simulink model "fadec_limit_logic"  (R2025b)
settings: Solver=FixedStepDiscrete  StartTime=0.0  StopTime=10.0  FixedStep=0.02  RelTol=1e-3

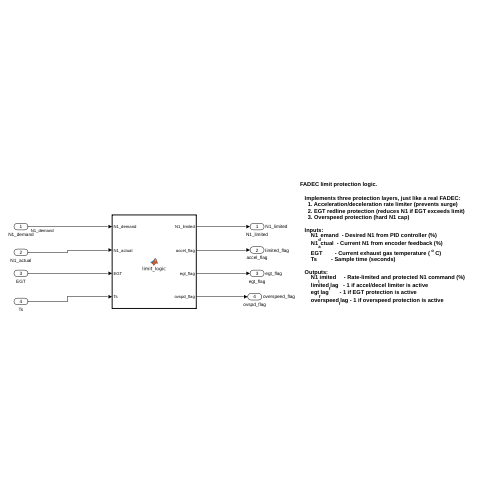
[thumbnail: Simulink's stored preview of the top-level diagram]
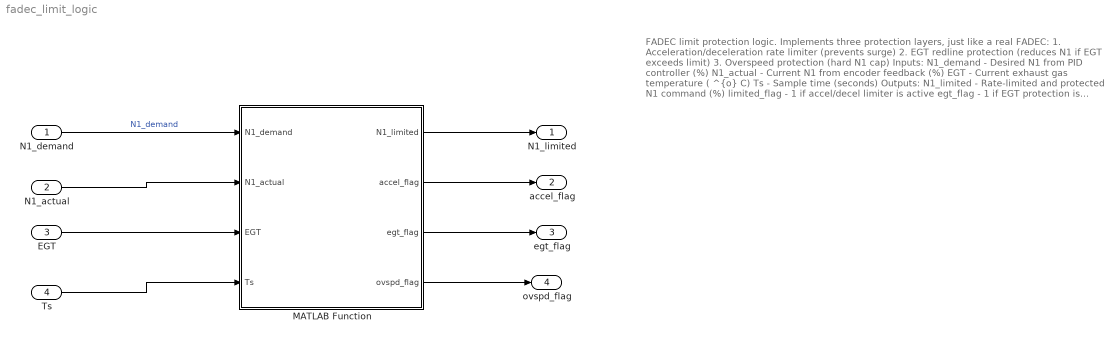
== system fadec_limit_logic ==
  note: FADEC limit protection logic.
      |
      |    Implements three protection layers, just like a real FADEC:
      |      1. Acceleration/deceleration rate limiter (prevents surge)
      |      2. EGT redline protection (reduces N1 if EGT exceeds limit)
      |      3. Overspeed protection (hard N1 cap)
      |
      |    Inputs:
      |        N1_demand  - Desired N1 from PID controller (%)
      |        N1_actual  - Current N1 from encoder feedback (%)
      |        EGT        - Current exhaust gas temperature ( ^{o} C)
      |        Ts         - Sample time (seconds)
      |
      |    Outputs:
      |        N1_limited     - Rate-limited and protected N1 command (%)
      |        limited_flag   - 1 if accel/decel limiter is active
      |        egt_flag       - 1 if EGT protection is active
      |        overspeed_flag - 1 if overspeed protection is active
  N1_demand : Inport
  N1_actual : Inport  Port=2
  EGT : Inport  Port=3
  Ts : Inport  Port=4
  MATLAB Function : MATLAB Function  TreatAsAtomicUnit=on
  N1_limited : Outport  SignalName=N1_limited
  accel_flag : Outport  Port=2  SignalName=limited_flag
  egt_flag : Outport  Port=3  SignalName=egt_flag
  ovspd_flag : Outport  Port=4  SignalName=overspeed_flag
  wires:
  N1_demand/1 -> MATLAB Function/1(N1_demand)  "N1_demand"
  N1_actual/1 -> MATLAB Function/2(N1_actual)
  EGT/1 -> MATLAB Function/3(EGT)
  Ts/1 -> MATLAB Function/4(Ts)
  MATLAB Function/4(ovspd_flag) -> ovspd_flag/1
  MATLAB Function/3(egt_flag) -> egt_flag/1
  MATLAB Function/2(accel_flag) -> accel_flag/1
  MATLAB Function/1(N1_limited) -> N1_limited/1

== matlab function fadec_limit_logic/MATLAB Function ==
  data: N1_demand input; N1_limited output; N1_actual input; EGT input; Ts input; accel_flag output; egt_flag output; ovspd_flag output
function [N1_limited, accel_flag, egt_flag, ovspd_flag] = ...
    limit_logic(N1_demand, N1_actual, EGT, Ts)

    persistent N1_prev;
    if isempty(N1_prev)
        N1_prev = 19.0;
    end

    MAX_ACCEL  = 8.0;
    MAX_DECEL  = 12.0;
    EGT_RED    = 1060;
    EGT_MARGIN = 30;
    N1_RED     = 104.0;

    % Bodyguard 1: acceleration limiter
    delta = N1_demand - N1_prev;
    max_up   =  MAX_ACCEL * Ts;
    max_down = -MAX_DECEL * Ts;
    delta_clamped = max(max_down, min(max_up, delta));
    N1_rate_limited = N1_prev + delta_clamped;
    accel_flag = double(abs(delta) > abs(delta_clamped) + 0.01);

    % Bodyguard 2: EGT protection
    egt_flag = double(0);
    N1_egt_limited = N1_rate_limited;
    if EGT > (EGT_RED - EGT_MARGIN)
        egt_excess = EGT - (EGT_RED - EGT_MARGIN);
        reduction = egt_excess * 0.5;
        N1_egt_limited = N1_rate_limited - reduction;
        N1_egt_limited = max(19.0, N1_egt_limited);
        egt_flag = double(1);
    end

    % Bodyguard 3: overspeed protection
    ovspd_flag = double(0);
    N1_final = N1_egt_limited;
    if N1_final > N1_RED
        N1_final = N1_RED;
        ovspd_flag = double(1);
    end

    N1_final = max(19.0, N1_final);
    N1_prev = N1_final;
    N1_limited = N1_final;
end
